simulink model "dynamiczny_ciagly"  (R2017b)
settings: Solver=VariableStepAuto  StartTime=0.0  StopTime=time  RelTol=1e-3
values from neighbouring files (symbols this model uses):
  alfa1 = -0.9    [params.m]
  alfa2 = 1.37    [params.m]
  alfa3 = -1.95    [params.m]
  alfa4 = 0.05    [params.m]
  DelayValue = 1    [params.m]
  K = 5    [params.m]
  StartDelay = 5    [params.m]
  StartValue = 0    [params.m]
  T1 = 10    [params.m]
  T2 = 6    [params.m]
settings Model: Creator=Tomek  LastModifiedBy=Tomek

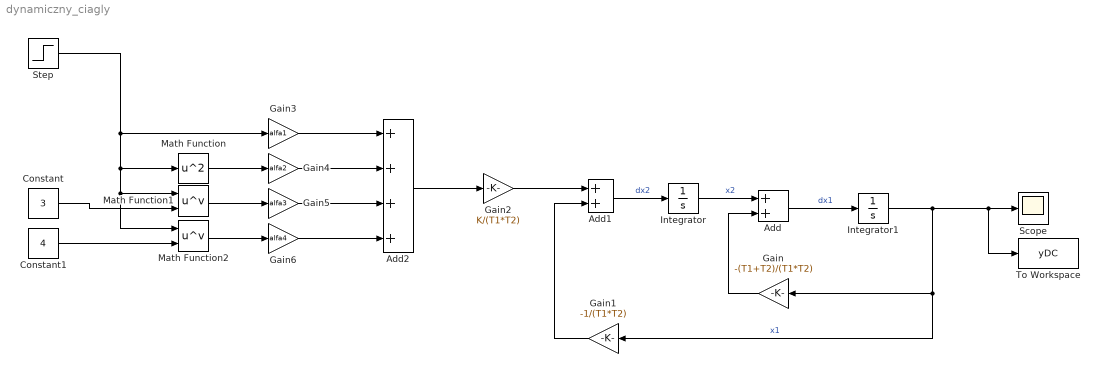
== system dynamiczny_ciagly ==
  Add : Sum
  Add1 : Sum
  Add2 : Sum  Inputs=++++
  Constant : Constant  Value=3
  Constant1 : Constant  Value=4
  Gain : Gain  Gain=-(T1+T2)/(T1*T2)
  Gain1 : Gain  Gain=-1/(T1*T2)
  Gain2 : Gain  Gain=K/(T1*T2)
  Gain3 : Gain  Gain=alfa1
  Gain4 : Gain  Gain=alfa2
  Gain5 : Gain  Gain=alfa3
  Gain6 : Gain  Gain=alfa4
  Integrator : Integrator
  Integrator1 : Integrator
  Math Function : Math  Operator=square  SaturateOnIntegerOverflow=on
  Math Function1 : Math  Operator=pow  SaturateOnIntegerOverflow=on
  Math Function2 : Math  Operator=pow  SaturateOnIntegerOverflow=on
  Scope : Scope
  Step : Step  Time=StartDelay  Before=StartValue  After=DelayValue  SampleTime=0
  To Workspace : ToWorkspace  VariableName=yDC  SaveFormat=Timeseries  SampleTime=-1
  wires:
  Integrator1/1 -> Gain1/1, Gain/1, To Workspace/1, Scope/1  "x1"
  Integrator/1 -> Add/1  "x2"
  Add1/1 -> Integrator/1  "dx2"
  Add/1 -> Integrator1/1  "dx1"
  Gain/1 -> Add/2
  Gain1/1 -> Add1/2
  Gain2/1 -> Add1/1
  Add2/1 -> Gain2/1
  Gain3/1 -> Add2/1
  Gain4/1 -> Add2/2
  Gain5/1 -> Add2/3
  Gain6/1 -> Add2/4
  Math Function/1 -> Gain4/1
  Math Function1/1 -> Gain5/1
  Math Function2/1 -> Gain6/1
  Step/1 -> Math Function2/1, Math Function1/1, Math Function/1, Gain3/1
  Constant/1 -> Math Function1/2
  Constant1/1 -> Math Function2/2
